simulink model "Sumpners"  (R2020a)
settings: Solver=VariableStepAuto  StartTime=0.0  StopTime=10.0  RelTol=1e-3
libraries: powerlib x9, powerlib_meascontrol x8, eePowerMeasurement x2
settings Model: Creator=ABHISHEK PRASAD  LastModifiedBy=ABHISHEK PRASAD

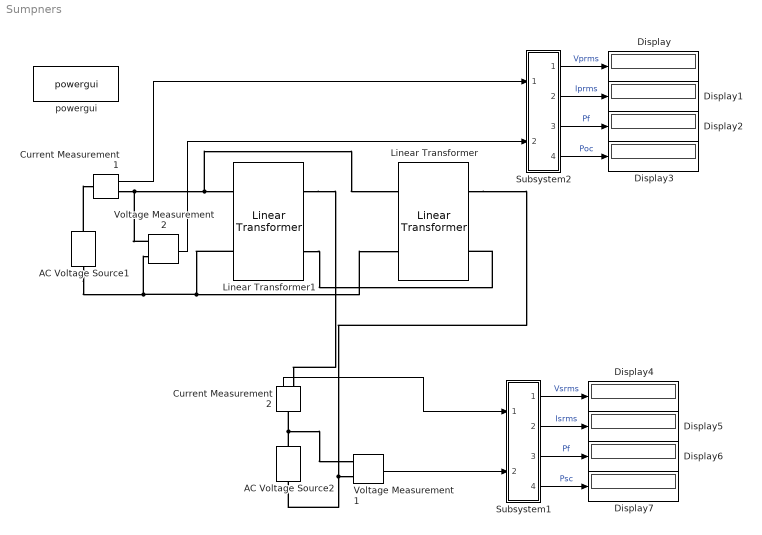
== system Sumpners ==
  AC Voltage Source1 : powerlib/Electrical Sources/AC Voltage Source  Amplitude=2400*1.414  Phase=0  Frequency=50  SampleTime=0  Measurements=Voltage  BusType=swing  Pref=10e3  Qref=0  Qmin=-inf  Qmax=+inf
  AC Voltage Source2 : powerlib/Electrical Sources/AC Voltage Source  Amplitude=10.4*1.414  Phase=0  Frequency=50  SampleTime=0  Measurements=Voltage  BusType=swing  Pref=10e3  Qref=0  Qmin=-inf  Qmax=+inf
  Current Measurement1 : powerlib/Measurements/Current Measurement  PhasorSimulation=off  OutputType=Complex  PSBequivalent=0
  Current Measurement2 : powerlib/Measurements/Current Measurement  PhasorSimulation=off  OutputType=Complex  PSBequivalent=0
  Display{,1..7} (8 alike) : Display
  Linear Transformer : powerlib/Elements/Linear Transformer  UNITS=SI  NominalPower=[ 50000 50 ]  winding1=[2400 0.7488 0.00319]  winding2=[240 0.007488 0.0000319]  ThreeWindings=off  winding3=[3.15e+05 3969 505.35]  RmLm=[33391 15.9409]  Measurements=None  DataType=on
  Linear Transformer1 : powerlib/Elements/Linear Transformer  UNITS=SI  NominalPower=[ 50000 50 ]  winding1=[2400 0.7488 0.00319]  winding2=[240 0.007488 0.0000319]  ThreeWindings=off  winding3=[3.15e+05 3969 505.35]  RmLm=[33391 15.9409]  Measurements=None  DataType=on
  Subsystem1 : Subsystem
  Subsystem2 : Subsystem
  Voltage Measurement1 : powerlib/Measurements/Voltage Measurement  PhasorSimulation=off  OutputType=Complex  PSBequivalent=0
  Voltage Measurement2 : powerlib/Measurements/Voltage Measurement  PhasorSimulation=off  OutputType=Complex  PSBequivalent=0
  powergui : powerlib/powergui  Priority=1  SimulationMode=Discrete  SampleTime=5e-4  frequency=50  Iterations=50  frequencyindice=50  Pbase=100e6  ErrMax=1e-4  UnitsV=kV  UnitsW=MW  buscounter=0  FunctionMessages=off  echomessages=off  EnableUseOfTLC=off  CurrentSourceSwitches=off  DisableSnubberDevices=off  DisableRonSwitches=off  DisableVfSwitches=off  DisplayEquations=off  AutomaticDiscreteSolvers=off  SolverType=Tustin/Backward Euler (TBE)  Interpol=off  ExternalGateDelay=off  methode=off  Ts=100  x0status=blocks  SPID=on  SwTol=0  HookPort=off  NonlinearTolerance=0  nMaxIteration=15  ContinueOnMaxIteration=off  RestoreLinks=warning  ResistiveCurrentMeasurement=off  Frange=[0:2:500]  Ylog=off  Xlog=on  ShowGrid=off  save=off  variable=ZData  structure=0  ZoomFFT=off  StartTime=0.0  cycles=1  DisplayStyle=1  fundamental=60  FreqAxis=off  MaxFrequency=1000  frequencyindicesteady=1  RmsSteady=1  display=off
  wires:
  Current Measurement1/1 -> Subsystem2/1(In1)
  Voltage Measurement2/1 -> Subsystem2/2(In2)
  Subsystem2/2(Out2) -> Display1/1  "Iprms"
  Subsystem2/3(Out3) -> Display2/1  "Pf"
  Subsystem2/4(Out4) -> Display3/1  "Poc"
  Subsystem2/1(Out1) -> Display/1  "Vprms"
  Subsystem1/1(Out1) -> Display4/1  "Vsrms"
  Subsystem1/4(Out4) -> Display7/1  "Psc"
  Subsystem1/3(Out3) -> Display6/1  "Pf"
  Subsystem1/2(Out2) -> Display5/1  "Isrms"
  Voltage Measurement1/1 -> Subsystem1/2(In2)
  Current Measurement2/1 -> Subsystem1/1(In1)
  connections:
  AC Voltage Source1/RConn1 -- Current Measurement1/LConn1
  Current Measurement1/RConn1 -- Voltage Measurement2/LConn1 -- Linear Transformer/LConn1 -- Linear Transformer1/LConn1
  AC Voltage Source1/LConn1 -- Linear Transformer/LConn2 -- Linear Transformer1/LConn2 -- Voltage Measurement2/LConn2
  AC Voltage Source2/RConn1 -- Voltage Measurement1/LConn1 -- Current Measurement2/LConn1
  Linear Transformer1/RConn2 -- Linear Transformer/RConn2
  Linear Transformer1/RConn1 -- Current Measurement2/RConn1
  Linear Transformer/RConn1 -- AC Voltage Source2/LConn1 -- Voltage Measurement1/LConn2

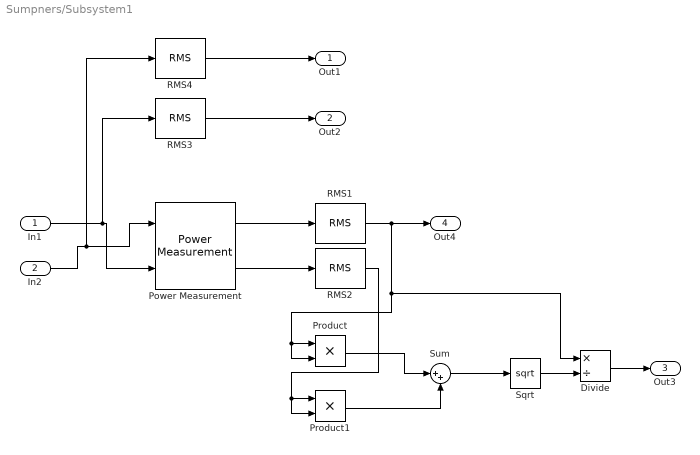
== system Sumpners/Subsystem1 ==
  In1 : Inport
  In2 : Inport  Port=2
  Divide : Product  Inputs=*/
  Power Measurement : eePowerMeasurement/Power Measurement  LabelModeActiveChoice=Continuous  F=50  K=[1]  Ts=0
      settings: SourceProductBaseCode=PS
  Product : Product
  Product1 : Product
  RMS{1..4} (4 alike) : powerlib_meascontrol/Measurements/RMS  TrueRMS=on  Freq=50  RMSInit=0  Ts=0
  Sqrt : Sqrt  SaturateOnIntegerOverflow=on
  Sum : Sum  Inputs=|++
  Out1 : Outport
  Out2 : Outport  Port=2
  Out3 : Outport  Port=3
  Out4 : Outport  Port=4
  wires:
  Divide/1 -> Out3/1
  Sqrt/1 -> Divide/2
  Sum/1 -> Sqrt/1
  Product1/1 -> Sum/2
  Product/1 -> Sum/1
  RMS2/1 -> Product1/2, Product1/1
  Power Measurement/2 -> RMS2/1
  RMS1/1 -> Out4/1, Product/1, Product/2, Divide/1
  RMS3/1 -> Out2/1
  RMS4/1 -> Out1/1
  Power Measurement/1 -> RMS1/1
  In2/1 -> Power Measurement/1, RMS4/1
  In1/1 -> Power Measurement/2, RMS3/1

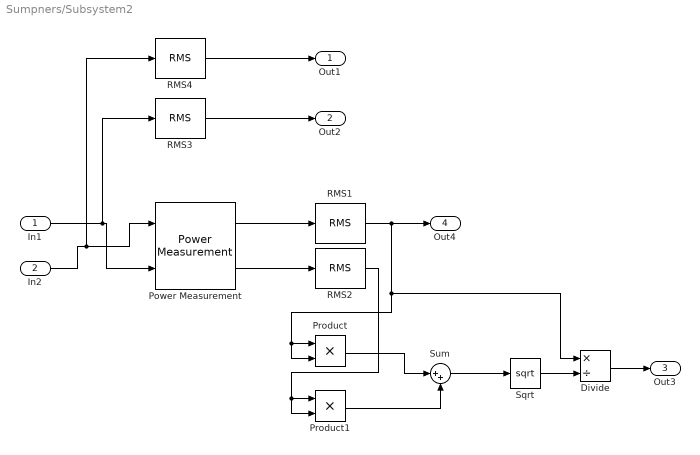
== system Sumpners/Subsystem2 ==
  In1 : Inport
  In2 : Inport  Port=2
  Divide : Product  Inputs=*/
  Power Measurement : eePowerMeasurement/Power Measurement  LabelModeActiveChoice=Continuous  F=50  K=[1]  Ts=0
      settings: SourceProductBaseCode=PS
  Product : Product
  Product1 : Product
  RMS{1..4} (4 alike) : powerlib_meascontrol/Measurements/RMS  TrueRMS=on  Freq=50  RMSInit=0  Ts=0
  Sqrt : Sqrt  SaturateOnIntegerOverflow=on
  Sum : Sum  Inputs=|++
  Out1 : Outport
  Out2 : Outport  Port=2
  Out3 : Outport  Port=3
  Out4 : Outport  Port=4
  wires:
  In1/1 -> RMS3/1, Power Measurement/2
  In2/1 -> RMS4/1, Power Measurement/1
  Power Measurement/1 -> RMS1/1
  RMS4/1 -> Out1/1
  RMS3/1 -> Out2/1
  RMS1/1 -> Divide/1, Product/2, Product/1, Out4/1
  Power Measurement/2 -> RMS2/1
  RMS2/1 -> Product1/1, Product1/2
  Product/1 -> Sum/1
  Product1/1 -> Sum/2
  Sum/1 -> Sqrt/1
  Sqrt/1 -> Divide/2
  Divide/1 -> Out3/1
